simulink model "Inverse_Dynamic_model"  (R2023a)
settings: Solver=VariableStepAuto  StartTime=0.0  StopTime=10  RelTol=1e-3
StopFcn:
  | clc
  | nL=7;
  | t=Tau.time;
  | Taun=Tau.signals.values;
  | for i=1:nL
  |     figure(i)
  | plot(t,Taun(:,i),'b-','LineWidth',2)
  | xlabel('time(s)')
  | ylabel(['\tau_',num2str(i),'(N.m)'])
  | grid
  | end
settings Model: Creator=HJokar  LastModifiedBy=pc
settings SolverCC: AlgebraicLoopSolver=TrustRegion
settings DataIOCC: ReturnWorkspaceOutputs=off
settings DebuggingCC: UnconnectedInputMsg=warning  UnconnectedOutputMsg=warning  UnconnectedLineMsg=warning  ArithmeticOperatorsInVariantConditions=warning
settings ModelReferenceCC: EnableRefExpFcnMdlSchedulingChecks=on
settings SFSimCC: CustomCodeUndefinedFunction=UseInterfaceOnly

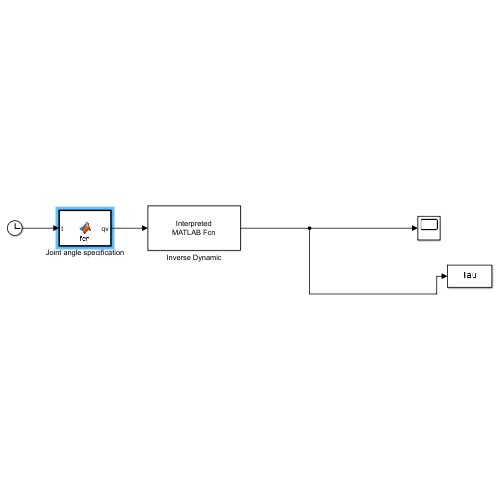
[thumbnail: Simulink's stored preview of the top-level diagram]
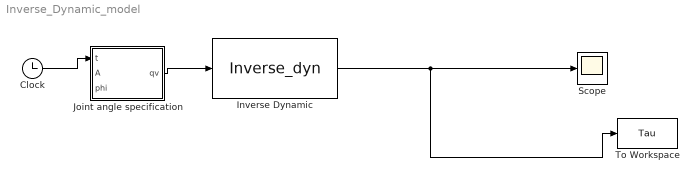
== system Inverse_Dynamic_model ==
  Clock : Clock
  Inverse Dynamic : MATLABFcn  MATLABFcn=Inverse_dyn  OutputSignalType=real
  Joint angle specification : MATLAB Function  TreatAsAtomicUnit=on
  Scope : Scope
  To Workspace : ToWorkspace  VariableName=Tau  SaveFormat=Structure With Time  SampleTime=-1
  wires:
  Inverse Dynamic/1 -> Scope/1, To Workspace/1
  Clock/1 -> Joint angle specification/1(t)
  Joint angle specification/1(qv) -> Inverse Dynamic/1

== matlab function Inverse_Dynamic_model/Joint angle specification ==
  data: qv output; t input; A input; phi input
function qv = fcn(t, A, phi)
    % Defines joint angles, velocities, and accelerations as sinusoidal functions of time.
    % Input: 
    %   t - Time (scalar, seconds)
    %   A - Amplitudes for each joint (7x1 vector, optional, default: [1, 0.5, 0.3, 0.2, 0.1, 0.05, 0])
    %   phi - Phase shifts for each joint (7x1 vector, optional, default: zeros(7,1))
    % Output: qv - [q; qd; qdd] (21x1 vector: angles, velocities, accelerations)

    % Default amplitudes (rad) for interesting variation
    if nargin < 2 || isempty(A)
        A = [1, 0.5, 0.3, 0.2, 0.1, 0.05, 0]'; % Joint 1 has largest amplitude, Joint 7 is static
    end

    % Default phase shifts (rad) for staggered motion
    if nargin < 3 || isempty(phi)
        phi = zeros(7, 1); % No phase shift by default
    end

    % Frequencies (rad/s) for each joint to create diversity
    omega = [1, 1.5, 2, 2.5, 3, 3.5, 4]'; % Increasing frequency for each joint

    % Joint angles (rad)
    q = A .* sin(omega * t + phi);

    % Joint velocities (rad/s)
    qd = A .* omega .* cos(omega * t + phi);

    % Joint accelerations (rad/s^2)
    qdd = -A .* omega.^2 .* sin(omega * t + phi);

    % Combine into state vector
    qv = [q; qd; qdd];
end
